simulink model "bipedal_robot_buV2_4"  (R2020b)
settings: Solver=ode23  StartTime=0.0  StopTime=Tsim  MaxStep=0.01  RelTol=1e-3  AbsTol=1e-3  EnableMultiTasking=on
undefined symbols (not defined in the file): Base, ctrl_config, ctrl_data, g, LefAnklePitch, LefAnkleRoll, LefHipPitch, LefHipRoll, LefHipYaw, LefKnee, lleg_str, RigAnklePitch, RigAnkleRoll, RigHipPitch, RigHipRoll, RigHipYaw, RigKnee, rleg_str, sim_floor, Tfil, TG_test_type, total_mass, Ts, X, Y, Z
libraries: sm_lib x53, biped_lib x34, nesl_utility x9, robotmaniplib x5, simulink x1, Contact_Forces_Lib x1
(part 1 of 3)
settings Model: Creator=Andraž  LastModifiedBy=isclab
settings SolverCC: AutoScaleAbsTol=off  ZeroCrossAlgorithm=Adaptive
settings DataIOCC: LimitDataPoints=on  MaxDataPoints=10000
settings OptimizationCC: LifeSpan=inf
settings DebuggingCC: IgnoredZcDiagnostic=none  AllowSymbolicDim=off  SFUnexpectedBacktrackingDiag=warning  SFNoUnconditionalDefaultTransitionDiag=warning  SFExecutionAtInitializationDiag=none  ArithmeticOperatorsInVariantConditions=warning
settings SFSimCC: SimUseLocalCustomCode=off  CustomCodeUndefinedFunction=UseInterfaceOnly
settings RTWCC: RTWUseLocalCustomCode=off
settings CodeAppCC: StateflowObjectComments=on
settings GRTTargetCC: TargetLangStandard=C89/C90 (ANSI)
settings ConfigComp: CovMetricSettings=dw  CovSaveCumulativeToWorkspaceVar=on  CovSaveSingleToWorkspaceVar=on  CovExternalEMLEnable=off  CovSFcnEnable=off
settings SimscapeCC: SimscapeLogType=all  SimscapeLogSimulationStatistics=on  SimscapeLogDataHistory=10000
settings DiagnosticsConfigSet: SimMechanicsRigidlyBoundBlock=none  SimMechanicsJointTargetOverSpecification=none
settings ExplorerConfigSet: InternalSimMechanicsExplorerSettings="<ExplorerConfiguration><canonicalview>default</canonicalview><AnimationSetting><BasePlaybackSpeed>1.0</BasePlaybackSpeed><PlaybackSpeedFactor>1.0</PlaybackSpeedFactor></AnimationSetting><TilePanel><TileInfo><Tiles Columns=\"1\" Count=\"1\" Rows=\"1\"><Column Weight=\"1\"/><Row Weight=\"1\"/><Tile Height=\"1\" Width=\"1\" X=\"0\" Y=\"0\"/></Tiles></TileInfo><SceneInfo><SceneViewer><BGColor><R>0.921568632125854492</R><G>0.913725495338439941</G><B>0.929411768913269043</B></BGColor><Camera><DoPerspective>off</DoPerspective><Position><X>1.46613297561511291</X><Y>0.0453876523198907741</Y><Z>0.392041392879294182</Z></Position><Center><X>-5.43948861508880555e-08</X><Y>0.0453876523198907741</Y><Z>0.392041392879294182</Z></Center><Up><X>-0</X><Y>0</Y><Z>1</Z></Up><ViewLimDist>1</ViewLimDist><YLim>0.627694802072910396</YLim><XLim>0.478013733886293257</XLim></Camera></SceneViewer></SceneInfo></TilePanel><MechEditorPanel><Cameras/><GfxPanelCameraMap/><VideoCreator><PlaybackSpeedRatio>1.0</PlaybackSpeedRatio><FrameRate>30</FrameRate><VideoFormat>Motion JPEG AVI</VideoFormat><FrameSize>auto</FrameSize></VideoCreator></MechEditorPanel></ExplorerConfiguration>"

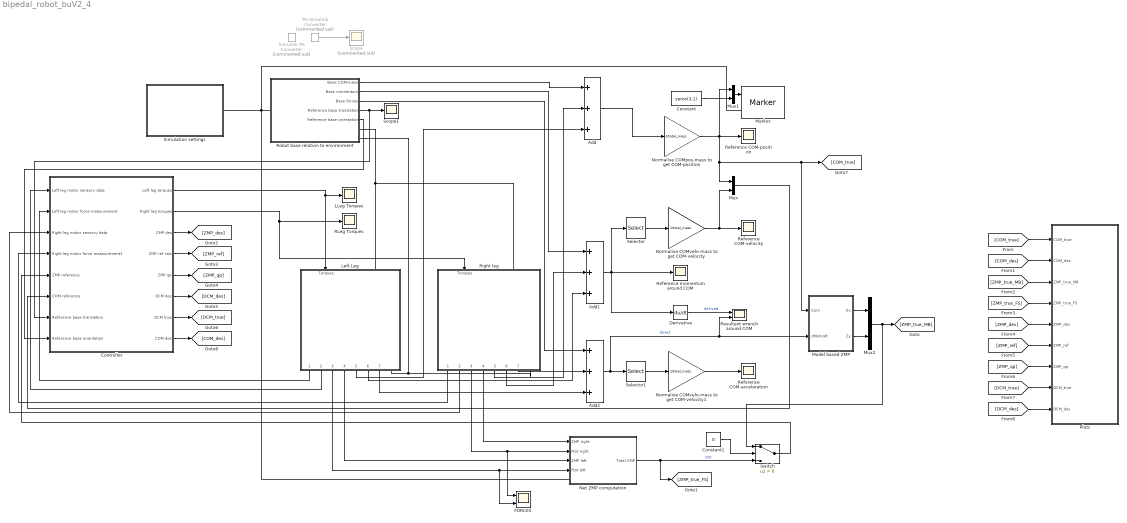
== system bipedal_robot_buV2_4 ==
  Add : Sum  Inputs=3
  Add1 : Sum  Inputs=3
  Add2 : Sum  Inputs=3
  Constant : Constant  Value=zeros(3,1)
  Constant1 : Constant  Value=0
  Controller : Subsystem
  Derivative : Derivative  CoefficientInTFapproximation=400
  FORCES : Scope  NumInputPorts=2
  LLeg Torques : Scope
  Left Leg : Subsystem
  Marker : biped_lib/Marker  colour=[1.0 0.8 0.4]
  Model based ZMP : Subsystem  mask{M=total_mass, g=g, Tfil=Tfil*0.5}
      mask prompts: M "Mass"; g "Gravity"; Tfil "Filtering constant"
  Mux : Mux  Inputs=2
  Mux1 : Mux  Inputs=2
  Mux2 : Mux  Inputs=2
  Net ZMP computation : Subsystem
  Normalise COMpos-mass to get COM-position : Gain  Gain=1/total_mass
  Normalise COMvelo-mass to get COM-velocity : Gain  Gain=1/total_mass
  Normalise COMvelo-mass to get COM-velocity1 : Gain  Gain=1/total_mass
  PS-Simulink Converter : nesl_utility/PS-Simulink Converter  Commented=on  PhysicalDomain=network_engine_domain  SubClassName=ps_output  LeftPortType=input  RightPortType=output  PseudoPeriodic=off  Frequencies=[]  Unit=inherit  AffineConversion=off
      settings: SourceProductName=Utilities
  Plots : Subsystem
  RLeg Torques : Scope
  Reference COM-acceleration : Scope
  Reference COM-position : Scope
  Reference COM-velocity : Scope
  Reference momentum around COM : Scope
  Resultant wrench around COM : Scope  NumInputPorts=2
  Right leg : Subsystem
  Robot base relation to environment : Subsystem
  Scope : Scope  Commented=on
  Scope1 : Scope
  Selector : Selector  InputPortWidth=6  IndexOptions=Index vector (dialog)  Indices=[1 2 3]  OutputSizes=1
  Selector1 : Selector  InputPortWidth=6  IndexOptions=Index vector (dialog)  Indices=[1 2 3]  OutputSizes=1
  Simulation settings : Subsystem
  Simulink-PS Converter : nesl_utility/Simulink-PS Converter  Commented=on  PhysicalDomain=network_engine_domain  SubClassName=ps_input  LeftPortType=input  RightPortType=output  PseudoPeriodic=off  Frequencies=[]  NoiseDistribution=none  NoiseParameters=[]  Unit=1  AffineConversion=off  FilteringAndDerivatives=provide  SimscapeFilterOrder=1  InputFilterTimeConstant=0.001  UdotUserProvided=0
      settings: SourceProductName=Utilities
  Switch : Switch  Criteria=u2 > Threshold
  wires:
  PS-Simulink Converter/1 -> Scope/1
  Controller/1(Left leg torques) -> Left Leg/1(Torques), LLeg Torques/1
  Controller/2(Right leg torques) -> Right leg/1(Torques), RLeg Torques/1
  Right leg/1(Contact data) -> Controller/4(Right leg motor force measurement1)
  Right leg/2(Motor sensory data) -> Controller/3(Right leg motor sensory data)
  Left Leg/2(Motor sensory data) -> Controller/1(Left leg motor sensory data)
  Left Leg/1(Contact data) -> Controller/2(Left leg motor force measurement)
  Right leg/3(Total force) -> FORCES/1, Net ZMP computation/2(Ftot right)
  Left Leg/3(Total force) -> FORCES/2, Net ZMP computation/4(Ftot left)
  Right leg/4(Zero moment point) -> Net ZMP computation/1(ZMP right)
  Left Leg/4(Zero moment point) -> Net ZMP computation/3(ZMP left)
  Net ZMP computation/1(Total ZMP) -> [ZMP_true_FS], Switch/3  "zIst"
  Robot base relation to environment/1(Base COM-mass) -> Add/1
  Left Leg/5(Leg COM-mass) -> Add/3
  Right leg/5(Leg COM-mass) -> Add/2
  Add/1 -> Normalise COMpos-mass to get COM-position/1
  Add1/1 -> Derivative/1, Reference momentum around COM/1, Selector/1
  Robot base relation to environment/2(Base momentum) -> Add1/1
  Right leg/6(Leg momentum) -> Add1/2
  Left Leg/6(Leg momentum) -> Add1/3
  Derivative/1 -> Resultant wrench around COM/1  "derived"
  Selector/1 -> Normalise COMvelo-mass to get COM-velocity/1
  Normalise COMvelo-mass to get COM-velocity/1 -> Mux/2, Reference COM-velocity/1
  Robot base relation to environment/3(Base forces) -> Add2/1
  Right leg/7(Leg momentum1) -> Add2/2
  Left Leg/7(Leg momentum1) -> Add2/3
  Add2/1 -> Selector1/1, Resultant wrench around COM/2, Model based ZMP/2(dMom/dt)  "direct"
  Normalise COMvelo-mass to get COM-velocity1/1 -> Reference COM-acceleration/1
  Selector1/1 -> Normalise COMvelo-mass to get COM-velocity1/1
  Normalise COMpos-mass to get COM-position/1 -> Mux1/1, Mux/1, Model based ZMP/1(Com), [COM_true], Reference COM-position/1
  Mux/1 -> Controller/6(COM reference)
  Robot base relation to environment/5(Reference base orientation) -> Controller/8(Reference base orientation)
  Robot base relation to environment/4(Reference base translation) -> Scope1/1, Controller/7(Reference base translation)
  Mux1/1 -> Marker/1
  Constant/1 -> Mux1/2
  Model based ZMP/1(Zx) -> Mux2/1
  Model based ZMP/2(Zy) -> Mux2/2
  Mux2/1 -> [ZMP_true_MB], Switch/1
  Constant1/1 -> Switch/2
  Switch/1 -> Controller/5(ZMP reference)
  [COM_true] -> Plots/1(COM_true)
  [COM_des] -> Plots/2(COM_des)
  [ZMP_true_MB] -> Plots/3(ZMP_true_MB)
  [ZMP_true_FS] -> Plots/4(ZMP_true_FS)
  [ZMP_des] -> Plots/5(ZMP_des)
  [ZMP_ref] -> Plots/6(ZMP_ref)
  [ZMP_qp] -> Plots/7(ZMP_qp)
  [DCM_true] -> Plots/8(DCM_true)
  [DCM_des] -> Plots/9(DCM_des)
  Controller/3(ZMP des) -> [ZMP_des]
  Controller/4(ZMP ref calc) -> [ZMP_ref]
  Controller/5(ZMP qp) -> [ZMP_qp]
  Controller/6(DCM des) -> [DCM_des]
  Controller/7(DCM true) -> [DCM_true]
  Controller/8(COM des) -> [COM_des]
  connections:
  Right leg/RConn1 -- Left Leg/RConn1 -- Robot base relation to environment/RConn2
  Left Leg/LConn1 -- Robot base relation to environment/RConn1 -- Right leg/LConn1
  Robot base relation to environment/LConn1 -- Simulation settings/RConn1 -- Marker/LConn1 -- Net ZMP computation/LConn1

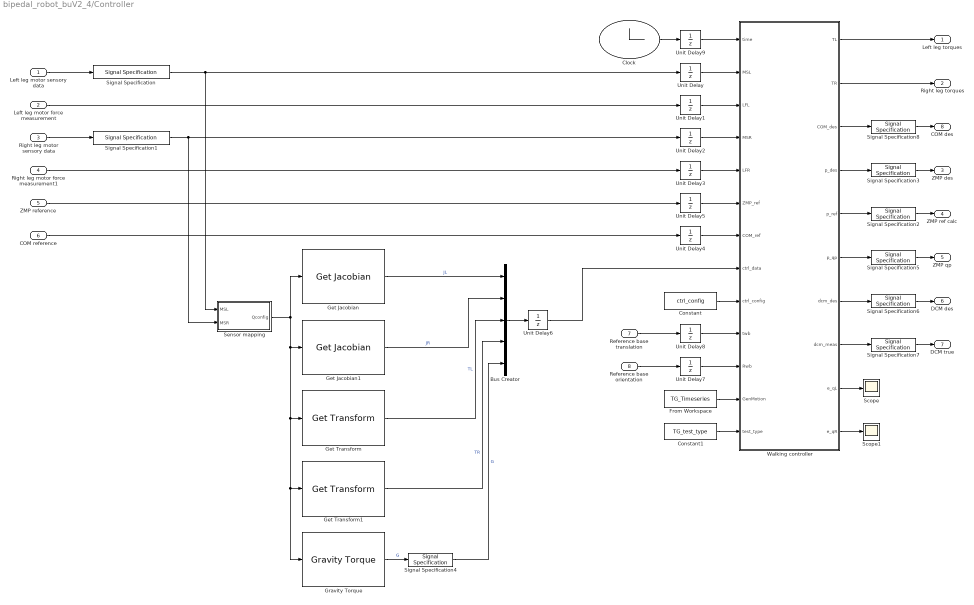
== system bipedal_robot_buV2_4/Controller ==
  Left leg motor sensory data : Inport
  Left leg motor force measurement : Inport  Port=2
  Right leg motor sensory data : Inport  Port=3
  Right leg motor force measurement1 : Inport  Port=4
  ZMP reference : Inport  Port=5
  COM reference : Inport  Port=6
  Reference base translation : Inport  Port=7
  Reference base orientation : Inport  Port=8
  Bus Creator : BusCreator  Inputs=5  OutDataTypeStr=Bus: ctrl_data_bus
  Clock : Clock
  Constant : Constant  Value=ctrl_config  OutDataTypeStr=Bus: ctrl_cfg_bus
  Constant1 : Constant  Value=TG_test_type
  From Workspace : FromWorkspace  VariableName=TG_Timeseries  SampleTime=Ts  OutputAfterFinalValue=Setting to zero
  Get Jacobian : robotmaniplib/Get Jacobian  RigidBodyTree=robot_model  EndEffector=EE_L  SimulateUsing=Code generation
      settings: SourceProductBaseCode=RO
  Get Jacobian1 : robotmaniplib/Get Jacobian  RigidBodyTree=robot_model  EndEffector=EE_R  SimulateUsing=Code generation
      settings: SourceProductBaseCode=RO
  Get Transform : robotmaniplib/Get Transform  RigidBodyTree=robot_model  SourceBody=FloBase  TargetBody=EE_L  SimulateUsing=Code generation
  Get Transform1 : robotmaniplib/Get Transform  RigidBodyTree=robot_model  SourceBody=FloBase  TargetBody=EE_R  SimulateUsing=Code generation
  Gravity Torque : robotmaniplib/Gravity Torque  RigidBodyTree=robot_model  SimulateUsing=Code generation
  Scope : Scope
  Scope1 : Scope
  Sensor mapping : MATLAB Function  TreatAsAtomicUnit=on
  Signal Specification : SignalSpecification  OutDataTypeStr=Bus: leg_str_bus
  Signal Specification1 : SignalSpecification  OutDataTypeStr=Bus: leg_str_bus
  Signal Specification{2..3,5..8} (6 alike) : SignalSpecification  Dimensions=2
  Signal Specification4 : SignalSpecification  Dimensions=[12,1]
  Unit Delay : UnitDelay  InitialCondition=lleg_str  SampleTime=Ts  HasFrameUpgradeWarning=on
  Unit Delay1 : UnitDelay  SampleTime=Ts  HasFrameUpgradeWarning=on
  Unit Delay2 : UnitDelay  InitialCondition=rleg_str  SampleTime=Ts  HasFrameUpgradeWarning=on
  Unit Delay3 : UnitDelay  SampleTime=Ts  HasFrameUpgradeWarning=on
  Unit Delay4 : UnitDelay  InitialCondition=zeros(6,1)  SampleTime=Ts  HasFrameUpgradeWarning=on
  Unit Delay5 : UnitDelay  InitialCondition=zeros(2,1)  SampleTime=Ts  HasFrameUpgradeWarning=on
  Unit Delay6 : UnitDelay  InitialCondition=ctrl_data  SampleTime=Ts  HasFrameUpgradeWarning=on
  Unit Delay7 : UnitDelay  InitialCondition=eye(3)  SampleTime=Ts  HasFrameUpgradeWarning=on
  Unit Delay8 : UnitDelay  InitialCondition=zeros(3,1)  SampleTime=Ts  HasFrameUpgradeWarning=on
  Unit Delay9 : UnitDelay  SampleTime=Ts  HasFrameUpgradeWarning=on
  Walking controller : MATLAB Function  TreatAsAtomicUnit=on
  Left leg torques : Outport
  Right leg torques : Outport  Port=2
  ZMP des : Outport  Port=3
  ZMP ref calc : Outport  Port=4
  ZMP qp : Outport  Port=5
  DCM des : Outport  Port=6
  DCM true : Outport  Port=7
  COM des : Outport  Port=8
  wires:
  Walking controller/1(TL) -> Left leg torques/1
  Walking controller/2(TR) -> Right leg torques/1
  Left leg motor sensory data/1 -> Signal Specification/1
  Left leg motor force measurement/1 -> Unit Delay1/1
  Right leg motor sensory data/1 -> Signal Specification1/1
  Right leg motor force measurement1/1 -> Unit Delay3/1
  Unit Delay/1 -> Walking controller/2(MSL)
  Unit Delay1/1 -> Walking controller/3(LFL)
  Unit Delay2/1 -> Walking controller/4(MSR)
  Unit Delay3/1 -> Walking controller/5(LFR)
  Signal Specification/1 -> Unit Delay/1, Sensor mapping/1(MSL)
  Signal Specification1/1 -> Unit Delay2/1, Sensor mapping/2(MSR)
  Unit Delay4/1 -> Walking controller/7(COM_ref)
  COM reference/1 -> Unit Delay4/1
  ZMP reference/1 -> Unit Delay5/1
  Unit Delay5/1 -> Walking controller/6(ZMP_ref)
  Get Jacobian/1 -> Bus Creator/1  "JL"
  Get Jacobian1/1 -> Bus Creator/2  "JR"
  Unit Delay6/1 -> Walking controller/8(ctrl_data)
  Constant/1 -> Walking controller/9(ctrl_config)
  Get Transform/1 -> Bus Creator/3  "TL"
  Get Transform1/1 -> Bus Creator/4  "TR"
  Bus Creator/1 -> Unit Delay6/1
  Reference base orientation/1 -> Unit Delay7/1
  Unit Delay7/1 -> Walking controller/11(Rwb)
  Reference base translation/1 -> Unit Delay8/1
  Unit Delay8/1 -> Walking controller/10(twb)
  Sensor mapping/1(Qconfig) -> Get Jacobian/1, Gravity Torque/1, Get Transform1/1, Get Transform/1, Get Jacobian1/1
  From Workspace/1 -> Walking controller/12(GenMotion)
  Unit Delay9/1 -> Walking controller/1(time)
  Clock/1 -> Unit Delay9/1
  Walking controller/5(p_ref) -> Signal Specification2/1
  Signal Specification2/1 -> ZMP ref calc/1
  Signal Specification3/1 -> ZMP des/1
  Walking controller/4(p_des) -> Signal Specification3/1
  Signal Specification4/1 -> Bus Creator/5  "G"
  Gravity Torque/1 -> Signal Specification4/1  "G"
  Constant1/1 -> Walking controller/13(test_type)
  Walking controller/9(e_qL) -> Scope/1
  Walking controller/10(e_qR) -> Scope1/1
  Signal Specification5/1 -> ZMP qp/1
  Walking controller/6(p_qp) -> Signal Specification5/1
  Signal Specification7/1 -> DCM true/1
  Signal Specification6/1 -> DCM des/1
  Walking controller/7(dcm_des) -> Signal Specification6/1
  Walking controller/8(dcm_meas) -> Signal Specification7/1
  Signal Specification8/1 -> COM des/1
  Walking controller/3(COM_des) -> Signal Specification8/1

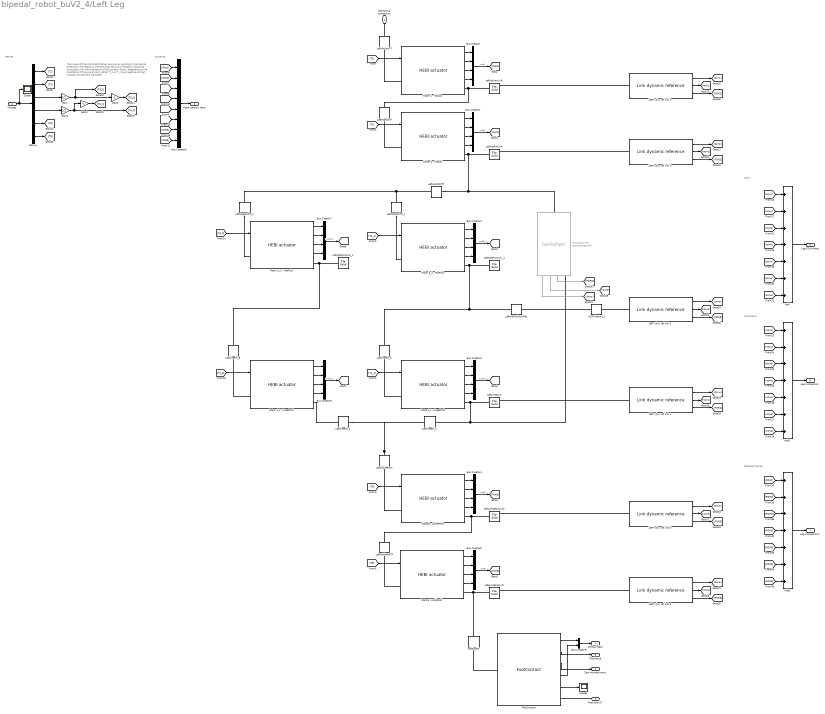
== system bipedal_robot_buV2_4/Left Leg ==
  note: Momentum
  note: COM
  note: OUTPUTS
  note: INPUTS
  note: The z-axes of the coordinate frames are always pointing in the
      | oposite directions. The reason is the following: the axis orientation
      | should be consistent with the orientation of the actuator frame. Depending on the orientation of the overall joint, either Ti_1 or Ti_2
      | are negative so that torques complement eachother
  note: Resultant forces
  Torques : Inport
  Add : Sum  Inputs=7
  Add1 : Sum  Inputs=7
  Add2 : Sum  Inputs=7
  Bus Creator{,1..5,7..8} (8 alike) : BusCreator  Inputs=4
  Bus Creator6 : BusCreator  Inputs=8  OutDataTypeStr=Bus: leg_str_bus
  Bus Creator9 : BusCreator  Inputs=2
  COM frame L3 : sm_lib/Frames and Transforms/Rigid Transform  TranslationMethod=Cartesian  TranslationStandardOffset=0  TranslationLengthUnit=m  TranslationStandardAxis=+Z  TranslationCartesianOffset=LefHipPitch.body.com  TranslationROffset=0  TranslationROffsetUnits=m  TranslationZOffset=0  TranslationZOffsetUnits=m  TranslationThetaOffset=0  TranslationThetaOffsetUnits=deg  RotationMethod=None  RotationAngleUnits=deg  RotationStandardAxis=+Z  RotationAngle=0.0  RotationArbitraryAxis=[0 0 1]  FollAlignAxisA=+X  BaseAlignAxisA=+Y  FollAlignAxisB=+Y  BaseAlignAxisB=+Z  RotationSequenceAxes=FollowerAxes  RotationSequence=XYX  RotationSequenceAngles=[0 0 0]  RotationSequenceAnglesUnits=deg  RotationMatrix=[1 0 0; 0 1 0; 0 0 1]
  Demux : Demux  Outputs=6
  FootContact : biped_lib/FootContact  SystemSampleTime=-1  VariantActivationTime=update diagram  Latency=0  AutoFrameSizeCalculation=off
  Gain : Gain  Gain=1/2
  Gain1 : Gain  Gain=1/2
  Gain2 : Gain  Gain=-1
  Gain3 : Gain  Gain=-1
  LEFT: dyn. ref. link 1 : biped_lib/Link dynamic reference  M=LefHipYaw.body.com  I=LefHipYaw.body.inertia
  LEFT: dyn. ref. link 2 : biped_lib/Link dynamic reference  M=LefHipRoll.body.mass  I=LefHipRoll.body.inertia
  LEFT: dyn. ref. link 3 : biped_lib/Link dynamic reference  M=LefHipPitch.body.mass  I=LefHipPitch.body.inertia
  LEFT: dyn. ref. link 4 : biped_lib/Link dynamic reference  M=LefKnee.body.mass  I=LefKnee.body.inertia
  LEFT: dyn. ref. link 5 : biped_lib/Link dynamic reference  M=LefAnklePitch.body.mass  I=LefAnklePitch.body.inertia
  LEFT: dyn. ref. link 6 : biped_lib/Link dynamic reference  M=LefAnkleRoll.body.mass  I=LefAnkleRoll.body.inertia
  LeftAnklePitch : sm_lib/Frames and Transforms/Rigid Transform  TranslationMethod=Cartesian  TranslationStandardOffset=0  TranslationLengthUnit=m  TranslationStandardAxis=+Z  TranslationCartesianOffset=LefAnklePitch.pos  TranslationROffset=0  TranslationROffsetUnits=m  TranslationZOffset=0  TranslationZOffsetUnits=m  TranslationThetaOffset=0  TranslationThetaOffsetUnits=deg  RotationMethod=RotationSequence  RotationAngleUnits=deg  RotationStandardAxis=+Z  RotationAngle=0.0  RotationArbitraryAxis=[0 0 1]  FollAlignAxisA=+X  BaseAlignAxisA=+Y  FollAlignAxisB=+Y  BaseAlignAxisB=+Z  RotationSequenceAxes=FollowerAxes  RotationSequence=XYZ  RotationSequenceAngles=LefAnklePitch.rot  RotationSequenceAnglesUnits=rad  RotationMatrix=[1 0 0; 0 1 0; 0 0 1]
  LeftAnklePitchLink : sm_lib/Body Elements/File Solid  ExtGeomFileName=Link5L_LR.stl  UnitType=Custom  ExtGeomFileUnits=mm  StepReaderType=HEX  ExportConvexHullGeometry=on  InertiaType=CalculateFromGeometry  Mass=LefAnklePitch.body.mass  MassUnits=kg  CenterOfMass=[0 0 0]  CenterOfMassUnits=m  MomentsOfInertia=[1 1 1]  MomentsOfInertiaUnits=kg*m^2  ProductsOfInertia=[0 0 0]  ProductsOfInertiaUnits=kg*m^2  BasedOnType=Mass  Density=1000  DensityUnits=kg/m^3  DoExposeReferenceFrame=on  SerializedFrames=<Frames><Frame><Id>Frame1</Id><Value><Name>COM</Name><Origin><Source>CenterOfMassFrame</Source><FeatureName></FeatureName></Origin><PrimaryAxis><DefinedDirection>+Z</DefinedDirection><Source>ReferenceFrame</Source><SourceDirection>+Z</SourceDirection><FeatureName></FeatureName></PrimaryAxis><SecondaryAxis><DefinedDirection>+X</DefinedDirection><Source>ReferenceFrame</Source><SourceDirection>+X</SourceDirection><FeatureName></FeatureName></SecondaryAxis></Value></Frame></Frames>  GraphicType=FromGeometry  MarkerShape=Sphere  MarkerSize=10  GraphicVisPropType=SimpleVisualProperties  GraphicDiffuseColor=[0.5 0.5 0.5]  GraphicSpecularColor=[0.5 0.5 0.5 1.0]  GraphicAmbientColor=[0.15 0.15 0.15 1.0]  GraphicEmissiveColor=[0.0 0.0 0.0 1.0]  GraphicShininess=75  GraphicOpacity=1.0
  LeftAnkleRollLink : sm_lib/Body Elements/File Solid  ExtGeomFileName=Link6_LR.stl  UnitType=Custom  ExtGeomFileUnits=mm  StepReaderType=HEX  ExportConvexHullGeometry=on  InertiaType=CalculateFromGeometry  Mass=LefAnkleRoll.body.mass  MassUnits=kg  CenterOfMass=[0 0 0]  CenterOfMassUnits=m  MomentsOfInertia=[1 1 1]  MomentsOfInertiaUnits=kg*m^2  ProductsOfInertia=[0 0 0]  ProductsOfInertiaUnits=kg*m^2  BasedOnType=Mass  Density=1000  DensityUnits=kg/m^3  DoExposeReferenceFrame=on  SerializedFrames=<Frames><Frame><Id>Frame1</Id><Value><Name>COM</Name><Origin><Source>CenterOfMassFrame</Source><FeatureName></FeatureName></Origin><PrimaryAxis><DefinedDirection>+Z</DefinedDirection><Source>ReferenceFrame</Source><SourceDirection>+Z</SourceDirection><FeatureName></FeatureName></PrimaryAxis><SecondaryAxis><DefinedDirection>+X</DefinedDirection><Source>ReferenceFrame</Source><SourceDirection>+X</SourceDirection><FeatureName></FeatureName></SecondaryAxis></Value></Frame></Frames>  GraphicType=FromGeometry  MarkerShape=Sphere  MarkerSize=10  GraphicVisPropType=SimpleVisualProperties  GraphicDiffuseColor=[0.5 0.5 0.5]  GraphicSpecularColor=[0.5 0.5 0.5 1.0]  GraphicAmbientColor=[0.15 0.15 0.15 1.0]  GraphicEmissiveColor=[0.0 0.0 0.0 1.0]  GraphicShininess=75  GraphicOpacity=1.0
  LeftAnkleRollTf : sm_lib/Frames and Transforms/Rigid Transform  TranslationMethod=Cartesian  TranslationStandardOffset=0  TranslationLengthUnit=m  TranslationStandardAxis=+Z  TranslationCartesianOffset=LefAnkleRoll.pos  TranslationROffset=0  TranslationROffsetUnits=m  TranslationZOffset=0  TranslationZOffsetUnits=m  TranslationThetaOffset=0  TranslationThetaOffsetUnits=deg  RotationMethod=RotationSequence  RotationAngleUnits=deg  RotationStandardAxis=+Z  RotationAngle=0.0  RotationArbitraryAxis=[0 0 1]  FollAlignAxisA=+Z  BaseAlignAxisA=+X  FollAlignAxisB=+Y  BaseAlignAxisB=+Y  RotationSequenceAxes=FollowerAxes  RotationSequence=XYZ  RotationSequenceAngles=LefAnkleRoll.rot  RotationSequenceAnglesUnits=rad  RotationMatrix=[1 0 0; 0 1 0; 0 0 1]
  LeftFootTf : sm_lib/Frames and Transforms/Rigid Transform  TranslationMethod=Cartesian  TranslationStandardOffset=0  TranslationLengthUnit=m  TranslationStandardAxis=+Z  TranslationCartesianOffset=LefFoot.pos  TranslationROffset=0  TranslationROffsetUnits=m  TranslationZOffset=0  TranslationZOffsetUnits=m  TranslationThetaOffset=0  TranslationThetaOffsetUnits=deg  RotationMethod=RotationSequence  RotationAngleUnits=deg  RotationStandardAxis=+Z  RotationAngle=0.0  RotationArbitraryAxis=[0 0 1]  FollAlignAxisA=+Z  BaseAlignAxisA=+Y  FollAlignAxisB=+X  BaseAlignAxisB=+X  RotationSequenceAxes=FollowerAxes  RotationSequence=XYZ  RotationSequenceAngles=LefFoot.rot  RotationSequenceAnglesUnits=rad  RotationMatrix=[1 0 0; 0 1 0; 0 0 1]
  LeftGasDamper : biped_lib/GasDamper  Commented=on  mech=LefDamper
  LeftHipPitchDynRef : sm_lib/Frames and Transforms/Rigid Transform  TranslationMethod=Cartesian  TranslationStandardOffset=0  TranslationLengthUnit=m  TranslationStandardAxis=+Z  TranslationCartesianOffset=-LefHipPitch.pos_1  TranslationROffset=0  TranslationROffsetUnits=m  TranslationZOffset=0  TranslationZOffsetUnits=m  TranslationThetaOffset=0  TranslationThetaOffsetUnits=deg  RotationMethod=None  RotationAngleUnits=deg  RotationStandardAxis=+Z  RotationAngle=0.0  RotationArbitraryAxis=[0 0 1]  FollAlignAxisA=+X  BaseAlignAxisA=+Y  FollAlignAxisB=+Y  BaseAlignAxisB=+Z  RotationSequenceAxes=FollowerAxes  RotationSequence=XYX  RotationSequenceAngles=[0 0 0]  RotationSequenceAnglesUnits=deg  RotationMatrix=[1 0 0; 0 1 0; 0 0 1]
  LeftHipPitchLink_1 : sm_lib/Body Elements/File Solid  ExtGeomFileName=Link3_LR.stl  UnitType=Custom  ExtGeomFileUnits=mm  StepReaderType=HEX  ExportConvexHullGeometry=on  InertiaType=CalculateFromGeometry  Mass=LefHipPitch.body.mass  MassUnits=kg  CenterOfMass=[0 0 0]  CenterOfMassUnits=m  MomentsOfInertia=[1 1 1]  MomentsOfInertiaUnits=kg*m^2  ProductsOfInertia=[0 0 0]  ProductsOfInertiaUnits=kg*m^2  BasedOnType=Mass  Density=1000  DensityUnits=kg/m^3  DoExposeReferenceFrame=on  SerializedFrames=<Frames/>  GraphicType=FromGeometry  MarkerShape=Sphere  MarkerSize=10  GraphicVisPropType=SimpleVisualProperties  GraphicDiffuseColor=[0.5 0.5 0.5]  GraphicSpecularColor=[0.5 0.5 0.5 1.0]  GraphicAmbientColor=[0.15 0.15 0.15 1.0]  GraphicEmissiveColor=[0.0 0.0 0.0 1.0]  GraphicShininess=75  GraphicOpacity=1.0
  LeftHipPitchLink_2 : sm_lib/Body Elements/File Solid  ExtGeomFileName=Link3_LR.stl  UnitType=Custom  ExtGeomFileUnits=mm  StepReaderType=HEX  ExportConvexHullGeometry=on  InertiaType=CalculateFromGeometry  Mass=LefHipPitch.body.mass  MassUnits=kg  CenterOfMass=[0 0 0]  CenterOfMassUnits=m  MomentsOfInertia=[1 1 1]  MomentsOfInertiaUnits=kg*m^2  ProductsOfInertia=[0 0 0]  ProductsOfInertiaUnits=kg*m^2  BasedOnType=Mass  Density=1000  DensityUnits=kg/m^3  DoExposeReferenceFrame=on  SerializedFrames=<Frames/>  GraphicType=FromGeometry  MarkerShape=Sphere  MarkerSize=10  GraphicVisPropType=SimpleVisualProperties  GraphicDiffuseColor=[0.5 0.5 0.5]  GraphicSpecularColor=[0.5 0.5 0.5 1.0]  GraphicAmbientColor=[0.15 0.15 0.15 1.0]  GraphicEmissiveColor=[0.0 0.0 0.0 1.0]  GraphicShininess=75  GraphicOpacity=1.0
  LeftHipPitchTf : sm_lib/Frames and Transforms/Rigid Transform  TranslationMethod=Cartesian  TranslationStandardOffset=0  TranslationLengthUnit=m  TranslationStandardAxis=+Z  TranslationCartesianOffset=LefHipPitch.pos  TranslationROffset=0  TranslationROffsetUnits=m  TranslationZOffset=0  TranslationZOffsetUnits=m  TranslationThetaOffset=0  TranslationThetaOffsetUnits=deg  RotationMethod=RotationSequence  RotationAngleUnits=deg  RotationStandardAxis=+Z  RotationAngle=0.0  RotationArbitraryAxis=[0 0 1]  FollAlignAxisA=+Z  BaseAlignAxisA=-X  FollAlignAxisB=+Y  BaseAlignAxisB=+Y  RotationSequenceAxes=FollowerAxes  RotationSequence=XYZ  RotationSequenceAngles=LefHipPitch.rot  RotationSequenceAnglesUnits=rad  RotationMatrix=[1 0 0; 0 1 0; 0 0 1]
  LeftHipPitchTf_1 : sm_lib/Frames and Transforms/Rigid Transform  TranslationMethod=Cartesian  TranslationStandardOffset=0  TranslationLengthUnit=m  TranslationStandardAxis=+Z  TranslationCartesianOffset=LefHipPitch.pos_1  TranslationROffset=0  TranslationROffsetUnits=m  TranslationZOffset=0  TranslationZOffsetUnits=m  TranslationThetaOffset=0  TranslationThetaOffsetUnits=deg  RotationMethod=RotationSequence  RotationAngleUnits=deg  RotationStandardAxis=+Z  RotationAngle=0.0  RotationArbitraryAxis=[0 0 1]  FollAlignAxisA=+X  BaseAlignAxisA=+Y  FollAlignAxisB=+Y  BaseAlignAxisB=+Z  RotationSequenceAxes=FollowerAxes  RotationSequence=XYZ  RotationSequenceAngles=LefHipPitch.rot_1  RotationSequenceAnglesUnits=rad  RotationMatrix=[1 0 0; 0 1 0; 0 0 1]
  LeftHipPitchTf_2 : sm_lib/Frames and Transforms/Rigid Transform  TranslationMethod=Cartesian  TranslationStandardOffset=0  TranslationLengthUnit=m  TranslationStandardAxis=+Z  TranslationCartesianOffset=LefHipPitch.pos_2  TranslationROffset=0  TranslationROffsetUnits=m  TranslationZOffset=0  TranslationZOffsetUnits=m  TranslationThetaOffset=0  TranslationThetaOffsetUnits=deg  RotationMethod=RotationSequence  RotationAngleUnits=deg  RotationStandardAxis=+Z  RotationAngle=0.0  RotationArbitraryAxis=[0 0 1]  FollAlignAxisA=+X  BaseAlignAxisA=+Y  FollAlignAxisB=+Y  BaseAlignAxisB=+Z  RotationSequenceAxes=FollowerAxes  RotationSequence=XYZ  RotationSequenceAngles=LefHipPitch.rot_2  RotationSequenceAnglesUnits=rad  RotationMatrix=[1 0 0; 0 1 0; 0 0 1]
  LeftHipRollLink : sm_lib/Body Elements/File Solid  ExtGeomFileName=Link2_LR.stl  UnitType=Custom  ExtGeomFileUnits=mm  StepReaderType=HEX  ExportConvexHullGeometry=on  InertiaType=CalculateFromGeometry  Mass=LefHipRoll.body.mass  MassUnits=kg  CenterOfMass=[0 0 0]  CenterOfMassUnits=m  MomentsOfInertia=[1 1 1]  MomentsOfInertiaUnits=kg*m^2  ProductsOfInertia=[0 0 0]  ProductsOfInertiaUnits=kg*m^2  BasedOnType=Mass  Density=1000  DensityUnits=kg/m^3  DoExposeReferenceFrame=on  SerializedFrames=<Frames><Frame><Id>Frame1</Id><Value><Name>COM</Name><Origin><Source>CenterOfMassFrame</Source><FeatureName></FeatureName></Origin><PrimaryAxis><DefinedDirection>+Z</DefinedDirection><Source>ReferenceFrame</Source><SourceDirection>+Z</SourceDirection><FeatureName></FeatureName></PrimaryAxis><SecondaryAxis><DefinedDirection>+X</DefinedDirection><Source>ReferenceFrame</Source><SourceDirection>+X</SourceDirection><FeatureName></FeatureName></SecondaryAxis></Value></Frame></Frames>  GraphicType=FromGeometry  MarkerShape=Sphere  MarkerSize=10  GraphicVisPropType=SimpleVisualProperties  GraphicDiffuseColor=[0.5 0.5 0.5]  GraphicSpecularColor=[0.5 0.5 0.5 1.0]  GraphicAmbientColor=[0.15 0.15 0.15 1.0]  GraphicEmissiveColor=[0.0 0.0 0.0 1.0]  GraphicShininess=75  GraphicOpacity=1.0
  LeftHipRollTf : sm_lib/Frames and Transforms/Rigid Transform  TranslationMethod=Cartesian  TranslationStandardOffset=0  TranslationLengthUnit=m  TranslationStandardAxis=+Z  TranslationCartesianOffset=LefHipRoll.pos  TranslationROffset=0  TranslationROffsetUnits=m  TranslationZOffset=0  TranslationZOffsetUnits=m  TranslationThetaOffset=0  TranslationThetaOffsetUnits=deg  RotationMethod=RotationSequence  RotationAngleUnits=deg  RotationStandardAxis=+Z  RotationAngle=0.0  RotationArbitraryAxis=[0 0 1]  FollAlignAxisA=+Z  BaseAlignAxisA=+Y  FollAlignAxisB=+X  BaseAlignAxisB=+X  RotationSequenceAxes=FollowerAxes  RotationSequence=XYZ  RotationSequenceAngles=LefHipRoll.rot  RotationSequenceAnglesUnits=rad  RotationMatrix=[1 0 0; 0 1 0; 0 0 1]
  LeftHipYawLink : sm_lib/Body Elements/File Solid  ExtGeomFileName=Link1L_LR.stl  UnitType=Custom  ExtGeomFileUnits=mm  StepReaderType=HEX  ExportConvexHullGeometry=on  InertiaType=CalculateFromGeometry  Mass=LefHipYaw.body.mass  MassUnits=kg  CenterOfMass=[0 0 0]  CenterOfMassUnits=m  MomentsOfInertia=[1 1 1]  MomentsOfInertiaUnits=kg*m^2  ProductsOfInertia=[0 0 0]  ProductsOfInertiaUnits=kg*m^2  BasedOnType=Mass  Density=1000  DensityUnits=kg/m^3  DoExposeReferenceFrame=on  SerializedFrames=<Frames><Frame><Id>Frame1</Id><Value><Name>COM</Name><Origin><Source>CenterOfMassFrame</Source><FeatureName></FeatureName></Origin><PrimaryAxis><DefinedDirection>+Z</DefinedDirection><Source>ReferenceFrame</Source><SourceDirection>+Z</SourceDirection><FeatureName></FeatureName></PrimaryAxis><SecondaryAxis><DefinedDirection>+X</DefinedDirection><Source>ReferenceFrame</Source><SourceDirection>+X</SourceDirection><FeatureName></FeatureName></SecondaryAxis></Value></Frame></Frames>  GraphicType=FromGeometry  MarkerShape=Sphere  MarkerSize=10  GraphicVisPropType=SimpleVisualProperties  GraphicDiffuseColor=[0.5 0.5 0.5]  GraphicSpecularColor=[0.5 0.5 0.5 1.0]  GraphicAmbientColor=[0.15 0.15 0.15 1.0]  GraphicEmissiveColor=[0.0 0.0 0.0 1.0]  GraphicShininess=75  GraphicOpacity=1.0
  LeftHipYawTf : sm_lib/Frames and Transforms/Rigid Transform  TranslationMethod=Cartesian  TranslationStandardOffset=0  TranslationLengthUnit=m  TranslationStandardAxis=+Z  TranslationCartesianOffset=LefHipYaw.pos  TranslationROffset=0  TranslationROffsetUnits=m  TranslationZOffset=0  TranslationZOffsetUnits=m  TranslationThetaOffset=0  TranslationThetaOffsetUnits=deg  RotationMethod=RotationSequence  RotationAngleUnits=deg  RotationStandardAxis=+Z  RotationAngle=0.0  RotationArbitraryAxis=[0 0 1]  FollAlignAxisA=+X  BaseAlignAxisA=+Y  FollAlignAxisB=+Y  BaseAlignAxisB=+Z  RotationSequenceAxes=FollowerAxes  RotationSequence=XYZ  RotationSequenceAngles=LefHipYaw.rot  RotationSequenceAnglesUnits=rad  RotationMatrix=[1 0 0; 0 1 0; 0 0 1]
  LeftKneeLink : sm_lib/Body Elements/File Solid  ExtGeomFileName=Link4_LR.stl  UnitType=Custom  ExtGeomFileUnits=mm  StepReaderType=HEX  ExportConvexHullGeometry=on  InertiaType=CalculateFromGeometry  Mass=LefKnee.body.mass  MassUnits=kg  CenterOfMass=[0 0 0]  CenterOfMassUnits=m  MomentsOfInertia=[1 1 1]  MomentsOfInertiaUnits=kg*m^2  ProductsOfInertia=[0 0 0]  ProductsOfInertiaUnits=kg*m^2  BasedOnType=Mass  Density=1000  DensityUnits=kg/m^3  DoExposeReferenceFrame=on  SerializedFrames=<Frames><Frame><Id>Frame1</Id><Value><Name>COM</Name><Origin><Source>CenterOfMassFrame</Source><FeatureName></FeatureName></Origin><PrimaryAxis><DefinedDirection>+Z</DefinedDirection><Source>ReferenceFrame</Source><SourceDirection>+Z</SourceDirection><FeatureName></FeatureName></PrimaryAxis><SecondaryAxis><DefinedDirection>+X</DefinedDirection><Source>ReferenceFrame</Source><SourceDirection>+X</SourceDirection><FeatureName></FeatureName></SecondaryAxis></Value></Frame></Frames>  GraphicType=FromGeometry  MarkerShape=Sphere  MarkerSize=10  GraphicVisPropType=SimpleVisualProperties  GraphicDiffuseColor=[0.5 0.5 0.5]  GraphicSpecularColor=[0.5 0.5 0.5 1.0]  GraphicAmbientColor=[0.15 0.15 0.15 1.0]  GraphicEmissiveColor=[0.0 0.0 0.0 1.0]  GraphicShininess=75  GraphicOpacity=1.0
  LeftKneeTf_1 : sm_lib/Frames and Transforms/Rigid Transform  TranslationMethod=Cartesian  TranslationStandardOffset=0  TranslationLengthUnit=m  TranslationStandardAxis=+Z  TranslationCartesianOffset=LefKnee.pos_1  TranslationROffset=0  TranslationROffsetUnits=m  TranslationZOffset=0  TranslationZOffsetUnits=m  TranslationThetaOffset=0  TranslationThetaOffsetUnits=deg  RotationMethod=RotationSequence  RotationAngleUnits=deg  RotationStandardAxis=+Z  RotationAngle=0.0  RotationArbitraryAxis=[0 0 1]  FollAlignAxisA=+X  BaseAlignAxisA=+Y  FollAlignAxisB=+Y  BaseAlignAxisB=+Z  RotationSequenceAxes=FollowerAxes  RotationSequence=XYZ  RotationSequenceAngles=LefKnee.rot_1  RotationSequenceAnglesUnits=rad  RotationMatrix=[1 0 0; 0 1 0; 0 0 1]
  LeftKneeTf_2 : sm_lib/Frames and Transforms/Rigid Transform  TranslationMethod=Cartesian  TranslationStandardOffset=0  TranslationLengthUnit=m  TranslationStandardAxis=+Z  TranslationCartesianOffset=LefKnee.pos_2  TranslationROffset=0  TranslationROffsetUnits=m  TranslationZOffset=0  TranslationZOffsetUnits=m  TranslationThetaOffset=0  TranslationThetaOffsetUnits=deg  RotationMethod=RotationSequence  RotationAngleUnits=deg  RotationStandardAxis=+Z  RotationAngle=0.0  RotationArbitraryAxis=[0 0 1]  FollAlignAxisA=+X  BaseAlignAxisA=+Y  FollAlignAxisB=+Y  BaseAlignAxisB=+Z  RotationSequenceAxes=FollowerAxes  RotationSequence=XYZ  RotationSequenceAngles=LefKnee.rot_2  RotationSequenceAnglesUnits=rad  RotationMatrix=[1 0 0; 0 1 0; 0 0 1]
  LeftKneeTf_A : sm_lib/Frames and Transforms/Rigid Transform  TranslationMethod=Cartesian  TranslationStandardOffset=0  TranslationLengthUnit=m  TranslationStandardAxis=+Z  TranslationCartesianOffset=LefKnee.pos  TranslationROffset=0  TranslationROffsetUnits=m  TranslationZOffset=0  TranslationZOffsetUnits=m  TranslationThetaOffset=0  TranslationThetaOffsetUnits=deg  RotationMethod=RotationSequence  RotationAngleUnits=deg  RotationStandardAxis=+Z  RotationAngle=0.0  RotationArbitraryAxis=[0 0 1]  FollAlignAxisA=+X  BaseAlignAxisA=+Y  FollAlignAxisB=+Y  BaseAlignAxisB=+Z  RotationSequenceAxes=FollowerAxes  RotationSequence=XYZ  RotationSequenceAngles=LefKnee.rot  RotationSequenceAnglesUnits=rad  RotationMatrix=[1 0 0; 0 1 0; 0 0 1]
  LeftKneeTf_B : sm_lib/Frames and Transforms/Rigid Transform  TranslationMethod=Cartesian  TranslationStandardOffset=0  TranslationLengthUnit=m  TranslationStandardAxis=+Z  TranslationCartesianOffset=LefKnee.pos  TranslationROffset=0  TranslationROffsetUnits=m  TranslationZOffset=0  TranslationZOffsetUnits=m  TranslationThetaOffset=0  TranslationThetaOffsetUnits=deg  RotationMethod=RotationSequence  RotationAngleUnits=deg  RotationStandardAxis=+Z  RotationAngle=0.0  RotationArbitraryAxis=[0 0 1]  FollAlignAxisA=+X  BaseAlignAxisA=+Y  FollAlignAxisB=+Y  BaseAlignAxisB=+Z  RotationSequenceAxes=FollowerAxes  RotationSequence=XYZ  RotationSequenceAngles=LefKnee.rot  RotationSequenceAnglesUnits=rad  RotationMatrix=[1 0 0; 0 1 0; 0 0 1]
  Motor 1 - HipYaw : biped_lib/HEBI actuator  Tmax=motor.X8.v16.Tmax  qinit=LefHipYaw.qinit  IMU=LefHipYaw.IMU
  Motor 2 - HipRoll : biped_lib/HEBI actuator  Tmax=motor.X8.v16.Tmax  qinit=LefHipRoll.qinit  IMU=LefHipRoll.IMU
  Motor 3_1 - HipPitch : biped_lib/HEBI actuator  Tmax=motor.X8.v16.Tmax  qinit=LefHipPitch.qinit_1  IMU=LefHipPitch.IMU_1
  Motor 3_2 - HipPitch : biped_lib/HEBI actuator  Tmax=motor.X8.v16.Tmax  qinit=LefHipPitch.qinit_2  IMU=LefHipPitch.IMU_2
  Motor 4_2 - KneePitch : biped_lib/HEBI actuator  Tmax=motor.X8.v16.Tmax  qinit=LefKnee.qinit_2  IMU=LefKnee.IMU_2
  Motor4_1 - KneePitch : biped_lib/HEBI actuator  Tmax=motor.X8.v16.Tmax  qinit=LefKnee.qinit_1  IMU=LefKnee.IMU_1
  Motor5 - AnklePitch : biped_lib/HEBI actuator  Tmax=motor.X8.v16.Tmax  qinit=LefAnklePitch.qinit  IMU=LefAnklePitch.IMU
  Motor6 - AnkleRoll : biped_lib/HEBI actuator  Tmax=motor.X8.v16.Tmax  qinit=LefAnkleRoll.qinit  IMU=LefAnkleRoll.IMU
  Scope : Scope
  Scope1 : Scope
  Mechanical connection : PMIOPort  Side=Left
  Foot sole CF : PMIOPort  Port=2  Side=Right
  Contact data : Outport
  Motor sensory data : Outport  Port=2
  Total force : Outport  Port=3
  Zero moment point : Outport  Port=4
  Leg COM-mass : Outport  Port=5
  Leg momentum : Outport  Port=6
  Leg momentum1 : Outport  Port=7
  wires:
  FootContact/1 -> Bus Creator9/1
  Motor 1 - HipYaw/4 -> Bus Creator/4
  Motor 1 - HipYaw/3 -> Bus Creator/3
  Motor 1 - HipYaw/2 -> Bus Creator/2
  Motor 1 - HipYaw/1 -> Bus Creator/1
  Motor 2 - HipRoll/1 -> Bus Creator1/1
  Motor 2 - HipRoll/2 -> Bus Creator1/2
  Motor 2 - HipRoll/3 -> Bus Creator1/3
  Motor 2 - HipRoll/4 -> Bus Creator1/4
  Motor 3_1 - HipPitch/2 -> Bus Creator2/2
  Motor 3_1 - HipPitch/1 -> Bus Creator2/1
  Motor 3_1 - HipPitch/3 -> Bus Creator2/3
  Motor 3_1 - HipPitch/4 -> Bus Creator2/4
  Motor4_1 - KneePitch/1 -> Bus Creator3/1
  Motor4_1 - KneePitch/2 -> Bus Creator3/2
  Motor4_1 - KneePitch/3 -> Bus Creator3/3
  Motor4_1 - KneePitch/4 -> Bus Creator3/4
  Motor5 - AnklePitch/1 -> Bus Creator4/1
  Motor5 - AnklePitch/2 -> Bus Creator4/2
  Motor5 - AnklePitch/3 -> Bus Creator4/3
  Motor5 - AnklePitch/4 -> Bus Creator4/4
  Motor6 - AnkleRoll/1 -> Bus Creator5/1
  Motor6 - AnkleRoll/2 -> Bus Creator5/2
  Motor6 - AnkleRoll/3 -> Bus Creator5/3
  Motor6 - AnkleRoll/4 -> Bus Creator5/4
  [T1] -> Motor 1 - HipYaw/1
  [T2] -> Motor 2 - HipRoll/1
  [T3_1] -> Motor 3_1 - HipPitch/1
  [T4_1] -> Motor4_1 - KneePitch/1
  [T5] -> Motor5 - AnklePitch/1
  [T6] -> Motor6 - AnkleRoll/1
  Bus Creator/1 -> [Mot1]  "mot1"
  Bus Creator1/1 -> [Mot2]  "mot2"
  Bus Creator2/1 -> [Mot3_1]  "mot3_1"
  Bus Creator3/1 -> [Mot4_1]  "mot4_1"
  Bus Creator4/1 -> [Mot5]  "mot5"
  Bus Creator5/1 -> [Mot6]  "mot6"
  Bus Creator6/1 -> Motor sensory data/1
  [Mot1] -> Bus Creator6/1
  [Mot2] -> Bus Creator6/2
  [Mot3_1] -> Bus Creator6/3
  [Mot4_1] -> Bus Creator6/5
  [Mot5] -> Bus Creator6/7
  [Mot6] -> Bus Creator6/8
  [Mot3_2] -> Bus Creator6/4
  [Mot4_2] -> Bus Creator6/6
  Bus Creator7/1 -> [Mot3_2]  "mot3_2"
  Motor 3_2 - HipPitch/2 -> Bus Creator7/2
  [T3_2] -> Motor 3_2 - HipPitch/1
  Motor 3_2 - HipPitch/1 -> Bus Creator7/1
  Motor 3_2 - HipPitch/3 -> Bus Creator7/3
  Motor 3_2 - HipPitch/4 -> Bus Creator7/4
  Bus Creator8/1 -> [Mot4_2]  "mot4_2"
  Motor 4_2 - KneePitch/3 -> Bus Creator8/3
  Motor 4_2 - KneePitch/2 -> Bus Creator8/2
  [T4_2] -> Motor 4_2 - KneePitch/1
  Motor 4_2 - KneePitch/4 -> Bus Creator8/4
  Motor 4_2 - KneePitch/1 -> Bus Creator8/1
  Torques/1 -> Scope/1, Demux/1
  Demux/1 -> [T1]
  Demux/2 -> [T2]
  Demux/3 -> Gain/1
  Gain/1 -> Gain2/1, [T3_1]
  Gain1/1 -> Gain3/1, [T4_2]
  Demux/4 -> Gain1/1
  Gain2/1 -> [T3_2]
  Gain3/1 -> [T4_1]
  Demux/5 -> [T5]
  Demux/6 -> [T6]
  FootContact/4 -> Bus Creator9/2
  Bus Creator9/1 -> Contact data/1
  FootContact/2 -> Total force/1
  FootContact/3 -> Zero moment point/1
  Add/1 -> Leg COM-mass/1
  Add1/1 -> Leg momentum/1
  LEFT: dyn. ref. link 1/1 -> [COM1]
  [COM1] -> Add/1
  LEFT: dyn. ref. link 2/1 -> [COM2]
  [COM2] -> Add/2
  LEFT: dyn. ref. link 3/1 -> [COM3]
  [COM3] -> Add/4
  [COM4] -> Add/5
  [COM5] -> Add/6
  [COM6] -> Add/7
  [COMD] -> Add/3
  LEFT: dyn. ref. link 4/1 -> [COM4]
  LEFT: dyn. ref. link 5/1 -> [COM5]
  LEFT: dyn. ref. link 6/1 -> [COM6]
  LeftGasDamper/1 -> [COMD]
  LEFT: dyn. ref. link 1/2 -> [MOM1]
  LEFT: dyn. ref. link 2/2 -> [MOM2]
  LEFT: dyn. ref. link 3/2 -> [MOM3]
  LEFT: dyn. ref. link 4/2 -> [MOM4]
  LEFT: dyn. ref. link 5/2 -> [MOM5]
  LEFT: dyn. ref. link 6/2 -> [MOM6]
  LeftGasDamper/2 -> [MOMD]
  [MOM3] -> Add1/4
  [MOM5] -> Add1/6
  [MOM1] -> Add1/1
  [MOM6] -> Add1/7
  [MOM2] -> Add1/2
  [MOMD] -> Add1/3
  [MOM4] -> Add1/5
  [FOR2] -> Add2/2
  [FOR4] -> Add2/5
  [FOR6] -> Add2/7
  [FOR3] -> Add2/4
  [FORD] -> Add2/3
  [FOR5] -> Add2/6
  Add2/1 -> Leg momentum1/1
  [FOR1] -> Add2/1
  LEFT: dyn. ref. link 1/3 -> [FOR1]
  LEFT: dyn. ref. link 2/3 -> [FOR2]
  LEFT: dyn. ref. link 3/3 -> [FOR3]
  LEFT: dyn. ref. link 4/3 -> [FOR4]
  LEFT: dyn. ref. link 5/3 -> [FOR5]
  LEFT: dyn. ref. link 6/3 -> [FOR6]
  LeftGasDamper/3 -> [FORD]
  FootContact/5 -> Scope1/1
  connections:
  LeftHipPitchTf/RConn1 -- LeftHipPitchTf_2/LConn1 -- LeftHipPitchTf_1/LConn1
  Motor6 - AnkleRoll/LConn1 -- LeftAnkleRollTf/RConn1
  Motor 2 - HipRoll/LConn1 -- LeftHipRollTf/RConn1
  LeftAnkleRollTf/LConn1 -- Motor5 - AnklePitch/RConn1 -- LeftAnklePitchLink/RConn1
  LeftHipPitchTf/LConn1 -- LeftGasDamper/LConn1 -- LeftHipRollLink/RConn1 -- Motor 2 - HipRoll/RConn1
  LeftFootTf/LConn1 -- LeftAnkleRollLink/RConn1 -- Motor6 - AnkleRoll/RConn1
  LeftKneeTf_A/LConn1 -- LeftHipPitchDynRef/LConn1 -- LeftHipPitchLink_1/RConn1 -- Motor 3_1 - HipPitch/RConn1
  LeftAnklePitch/RConn1 -- Motor5 - AnklePitch/LConn1
  Motor4_1 - KneePitch/LConn1 -- LeftKneeTf_A/RConn1
  LeftHipYawTf/RConn1 -- Motor 1 - HipYaw/LConn1
  LeftAnklePitch/LConn1 -- LeftKneeTf_1/RConn1 -- LeftKneeTf_2/RConn1
  FootContact/LConn1 -- LeftFootTf/RConn1
  LeftHipYawLink/RConn1 -- LeftHipRollTf/LConn1 -- Motor 1 - HipYaw/RConn1
  FootContact/RConn1 -- Foot sole CF/RConn1
  LeftHipYawTf/LConn1 -- Mechanical connection/RConn1
  LeftHipPitchTf_1/RConn1 -- Motor 3_1 - HipPitch/LConn1
  LeftHipPitchTf_2/RConn1 -- Motor 3_2 - HipPitch/LConn1
  LeftKneeTf_B/LConn1 -- LeftHipPitchLink_2/RConn1 -- Motor 3_2 - HipPitch/RConn1
  Motor 4_2 - KneePitch/RConn1 -- LeftKneeTf_2/LConn1
  Motor 4_2 - KneePitch/LConn1 -- LeftKneeTf_B/RConn1
  LeftKneeLink/RConn1 -- Motor4_1 - KneePitch/RConn1 -- LeftGasDamper/RConn1 -- LeftKneeTf_1/LConn1
  COM frame L3/LConn1 -- LeftHipPitchDynRef/RConn1
  LEFT: dyn. ref. link 1/LConn1 -- LeftHipYawLink/LConn1
  LEFT: dyn. ref. link 2/LConn1 -- LeftHipRollLink/LConn1
  LEFT: dyn. ref. link 3/LConn1 -- COM frame L3/RConn1
  LEFT: dyn. ref. link 4/LConn1 -- LeftKneeLink/LConn1
  LEFT: dyn. ref. link 5/LConn1 -- LeftAnklePitchLink/LConn1
  LEFT: dyn. ref. link 6/LConn1 -- LeftAnkleRollLink/LConn1

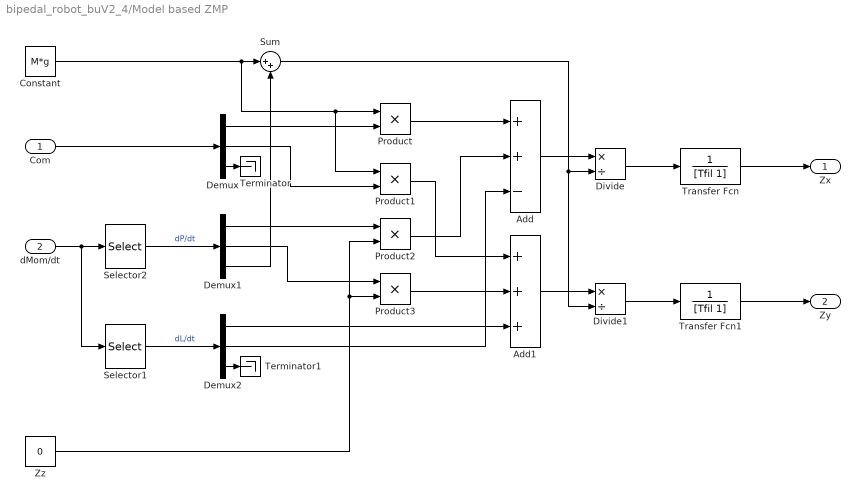
== system bipedal_robot_buV2_4/Model based ZMP ==
  Com : Inport
  dMom/dt : Inport  Port=2
  Add : Sum  Inputs=++-
  Add1 : Sum  Inputs=+++
  Constant : Constant  Value=M*g
  Demux : Demux  Outputs=3
  Demux1 : Demux  Outputs=3
  Demux2 : Demux  Outputs=3
  Divide : Product  Inputs=*/
  Divide1 : Product  Inputs=*/
  Product{,1..3} (4 alike) : Product
  Selector1 : Selector  InputPortWidth=6  IndexOptions=Index vector (dialog)  Indices=[4:6]  OutputSizes=1
  Selector2 : Selector  InputPortWidth=6  IndexOptions=Index vector (dialog)  Indices=[1:3]  OutputSizes=1
  Sum : Sum  Inputs=|++
  Terminator : Terminator
  Terminator1 : Terminator
  Transfer Fcn : TransferFcn  Denominator=[Tfil 1]
  Transfer Fcn1 : TransferFcn  Denominator=[Tfil 1]
  Zz : Constant  Value=0
  Zx : Outport
  Zy : Outport  Port=2
  wires:
  Com/1 -> Demux/1
  dMom/dt/1 -> Selector1/1, Selector2/1
  Selector1/1 -> Demux2/1  "dL/dt"
  Demux/1 -> Product/2
  Constant/1 -> Sum/1, Product1/1, Product/1
  Demux/2 -> Product1/2
  Demux1/1 -> Product2/1
  Zz/1 -> Product3/2, Product2/2
  Demux1/2 -> Product3/1
  Demux1/3 -> Sum/2
  Demux2/3 -> Terminator1/1
  Demux/3 -> Terminator/1
  Product/1 -> Add/1
  Product2/1 -> Add/2
  Demux2/2 -> Add/3
  Demux2/1 -> Add1/3
  Product3/1 -> Add1/2
  Product1/1 -> Add1/1
  Add/1 -> Divide/1
  Add1/1 -> Divide1/1
  Sum/1 -> Divide1/2, Divide/2
  Divide/1 -> Transfer Fcn/1
  Divide1/1 -> Transfer Fcn1/1
  Selector2/1 -> Demux1/1  "dP/dt"
  Transfer Fcn1/1 -> Zy/1
  Transfer Fcn/1 -> Zx/1
